simulink library "INT_APP_ChkSig"  (R2016b)
settings: Solver=VariableStepAuto  StartTime=0.0  StopTime=10.0  RelTol=1e-3
settings Model: Creator=xuxingpei  LastModifiedBy=xuxingpei

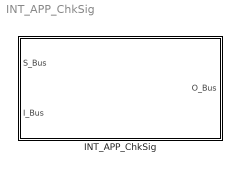
== system INT_APP_ChkSig ==
  INT_APP_ChkSig : Subsystem

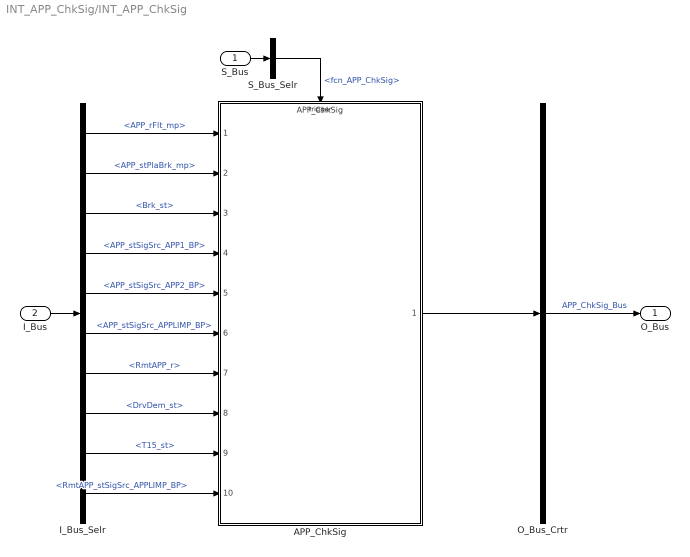
== system INT_APP_ChkSig/INT_APP_ChkSig ==
  S_Bus : Inport
  I_Bus : Inport  Port=2
  APP_ChkSig : ModelReference  ModelNameDialog=APP_ChkSig  SimulationMode=Normal  ModelReferenceVersion=1.57  TriggerPortName=function  TriggerPortTriggerType=function-call  TriggerPortStatesWhenEnabling=held
  I_Bus_Selr : BusSelector  OutputSignals=APP_rFlt_mp,APP_stPlaBrk_mp,Brk_st,APP_stSigSrc_APP1_BP,APP_stSigSrc_APP2_BP,APP_stSigSrc_APPLIMP_BP,RmtAPP_r,DrvDem_st,T15_st,RmtAPP_stSigSrc_APPLIMP_BP
  O_Bus_Crtr : BusCreator  Inputs=1
  S_Bus_Selr : BusSelector  OutputSignals=fcn_APP_ChkSig
  O_Bus : Outport
  wires:
  S_Bus_Selr/1 -> APP_ChkSig/Trigger  "<fcn_APP_ChkSig>"
  S_Bus/1 -> S_Bus_Selr/1
  I_Bus/1 -> I_Bus_Selr/1
  I_Bus_Selr/1 -> APP_ChkSig/1  "<APP_rFlt_mp>"
  I_Bus_Selr/2 -> APP_ChkSig/2  "<APP_stPlaBrk_mp>"
  I_Bus_Selr/3 -> APP_ChkSig/3  "<Brk_st>"
  I_Bus_Selr/4 -> APP_ChkSig/4  "<APP_stSigSrc_APP1_BP>"
  I_Bus_Selr/5 -> APP_ChkSig/5  "<APP_stSigSrc_APP2_BP>"
  I_Bus_Selr/6 -> APP_ChkSig/6  "<APP_stSigSrc_APPLIMP_BP>"
  I_Bus_Selr/7 -> APP_ChkSig/7  "<RmtAPP_r>"
  I_Bus_Selr/8 -> APP_ChkSig/8  "<DrvDem_st>"
  I_Bus_Selr/9 -> APP_ChkSig/9  "<T15_st>"
  I_Bus_Selr/10 -> APP_ChkSig/10  "<RmtAPP_stSigSrc_APPLIMP_BP>"
  O_Bus_Crtr/1 -> O_Bus/1  "APP_ChkSig_Bus"
  APP_ChkSig/1 -> O_Bus_Crtr/1
